simulink model "IEEE_religador"  (R2021b)
settings: Solver=ode23t  StartTime=0.0  StopTime=4  MaxStep=1e-4  RelTol=1e-3
undefined symbols (not defined in the file or in its folder): D1, Delta
libraries: spsThreePhasePISectionLineLib x36, spsThreePhaseVIMeasurementLib x34, spsSeriesRLCLoadLib x30, dsparch4 x24, spsSampleandHoldLib x24, spsNeutralLib x21, dspstat3 x20, spsPiSectionLineLib x15, spsLoadFlowBusLib x9, spsThreePhaseSeriesRLCLoadLib x8, spsThreePhaseFaultLib x7, spsThreePhaseBreakerLib x5
(part 1 of 2)
settings Model: SimulationMode=accelerator  Creator=Jamile-LARCA  LastModifiedBy=Ramayana
settings SolverCC: AlgebraicLoopSolver=TrustRegion
settings DataIOCC: ReturnWorkspaceOutputs=off
settings DebuggingCC: SFMachineParentedDataDiag=warning  ArithmeticOperatorsInVariantConditions=warning
settings SFSimCC: SimUseLocalCustomCode=off  CustomCodeUndefinedFunction=UseInterfaceOnly
settings RTWCC: RTWUseLocalCustomCode=off
settings CodeAppCC: StateflowObjectComments=on
settings SimscapeCC: SimscapeNormalizeSystem=off

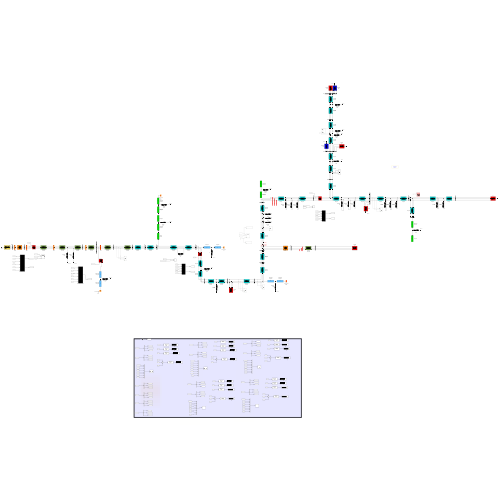
[thumbnail: Simulink's stored preview of the top-level diagram]
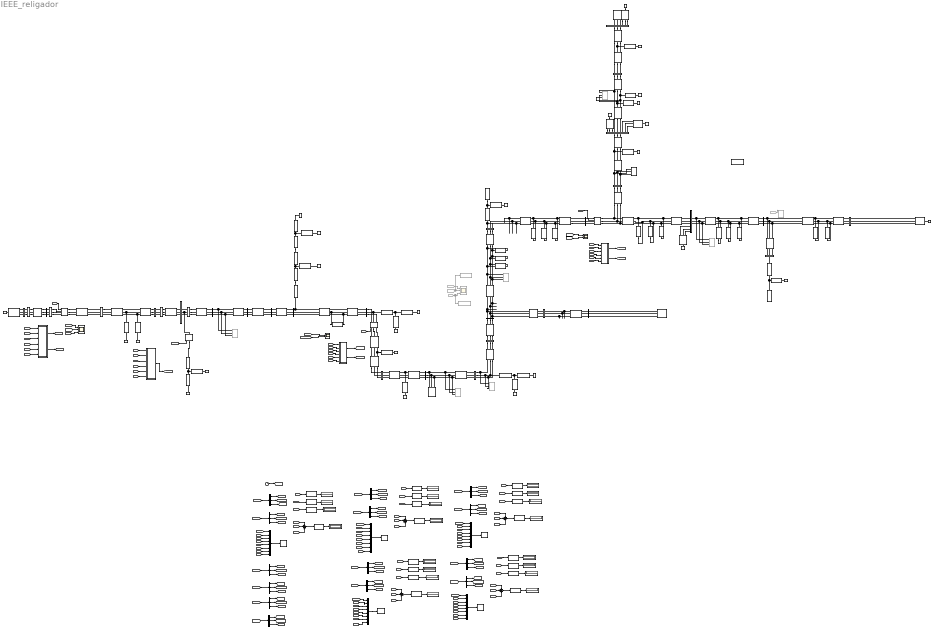
== system IEEE_religador ==
  note: 808
  note: Measurements
  " 816-824 D-I" : spsSeriesRLCLoadLib/Series RLC Load  LConnTagsString=a  RConnTagsString=__new0  NominalVoltage=24.9e3  NominalFrequency=60  ActivePower=5e3  InductivePower=2e3  CapacitivePower=0  Setx0=off  InitialVoltage=0  SetiL0=off  InitialCurrent=0  Measurements=None  LoadType=constant I
  " 824-826 Y-I" : spsSeriesRLCLoadLib/Series RLC Load  LConnTagsString=a  RConnTagsString=__new0  NominalVoltage=1.0156*14.376e3  NominalFrequency=60  ActivePower=40e3  InductivePower=20e3  CapacitivePower=0  Setx0=off  InitialVoltage=0  SetiL0=off  InitialCurrent=0  Measurements=None  LoadType=constant I
  " 828-830 Y-PQ" : spsSeriesRLCLoadLib/Series RLC Load  LConnTagsString=a  RConnTagsString=__new0  NominalVoltage=14.376e3  NominalFrequency=60  ActivePower=7e3  InductivePower=3e3  CapacitivePower=0  Setx0=off  InitialVoltage=0  SetiL0=off  InitialCurrent=0  Measurements=None  LoadType=constant PQ
  " 854-856 Y-PQ" : spsSeriesRLCLoadLib/Series RLC Load  LConnTagsString=a  RConnTagsString=__new0  NominalVoltage=0.9977*14.376e3  NominalFrequency=60  ActivePower=4e3  InductivePower=2e3  CapacitivePower=0  Setx0=off  InitialVoltage=0  SetiL0=off  InitialCurrent=0  Measurements=None  LoadType=constant PQ
  " L808-810a config 303 " : spsPiSectionLineLib/Pi Section Line  LConnTagsString=__new0  RConnTagsString=__new0  Phases=1  PiSections=1  Length=0.8845  Frequency=60  Resistance=1.7395  Inductance=2.4483e-3  Capacitance=6.9641e-9  Measurements=None  Measurements2=None
      settings: SourceProductBaseCode=PS
  " L808-810b config 303 " : spsPiSectionLineLib/Pi Section Line  LConnTagsString=__new0  RConnTagsString=__new0  Phases=1  PiSections=1  Length=0.8845  Frequency=60  Resistance=1.7395  Inductance=2.4483e-3  Capacitance=6.9641e-9  Measurements=None  Measurements2=None
      settings: SourceProductBaseCode=PS
  " L816-818 config 302" : spsPiSectionLineLib/Pi Section Line  LConnTagsString=__new0  RConnTagsString=__new0  Phases=1  PiSections=1  Length=0.521208  Frequency=60  Resistance=1.7395  Inductance=2.4483e-3  Capacitance=6.9641e-9  Measurements=None  Measurements2=None
      settings: SourceProductBaseCode=PS
  " L818-820a config 302" : spsPiSectionLineLib/Pi Section Line  LConnTagsString=__new0  RConnTagsString=__new0  Phases=1  PiSections=1  Length=7.3381  Frequency=60  Resistance=1.7395  Inductance=2.4483e-3  Capacitance=6.9641e-9  Measurements=None  Measurements2=None
      settings: SourceProductBaseCode=PS
  " L818-820b config 302" : spsPiSectionLineLib/Pi Section Line  LConnTagsString=__new0  RConnTagsString=__new0  Phases=1  PiSections=1  Length=7.3381  Frequency=60  Resistance=1.7395  Inductance=2.4483e-3  Capacitance=6.9641e-9  Measurements=None  Measurements2=None
      settings: SourceProductBaseCode=PS
  " L820-822a config 302" : spsPiSectionLineLib/Pi Section Line  LConnTagsString=__new0  RConnTagsString=__new0  Phases=1  PiSections=1  Length=2.0940  Frequency=60  Resistance=1.7395  Inductance=2.4483e-3  Capacitance=6.9641e-9  Measurements=None  Measurements2=None
      settings: SourceProductBaseCode=PS
  " L820-822b config 302" : spsPiSectionLineLib/Pi Section Line  LConnTagsString=__new0  RConnTagsString=__new0  Phases=1  PiSections=1  Length=2.0940  Frequency=60  Resistance=1.7395  Inductance=2.4483e-3  Capacitance=6.9641e-9  Measurements=None  Measurements2=None
      settings: SourceProductBaseCode=PS
  " L824-826a config 303 " : spsPiSectionLineLib/Pi Section Line  LConnTagsString=__new0  RConnTagsString=__new0  Phases=1  PiSections=1  Length=0.4618  Frequency=60  Resistance=1.7395  Inductance=2.4483e-3  Capacitance=6.9641e-9  Measurements=None  Measurements2=None
      settings: SourceProductBaseCode=PS
  " L824-826b config 303 " : spsPiSectionLineLib/Pi Section Line  LConnTagsString=__new0  RConnTagsString=__new0  Phases=1  PiSections=1  Length=0.4618  Frequency=60  Resistance=1.7395  Inductance=2.4483e-3  Capacitance=6.9641e-9  Measurements=None  Measurements2=None
      settings: SourceProductBaseCode=PS
  " L854-856a config 303 " : spsPiSectionLineLib/Pi Section Line  LConnTagsString=__new0  RConnTagsString=__new0  Phases=1  PiSections=1  Length=3.5555  Frequency=60  Resistance=1.7395  Inductance=2.4483e-3  Capacitance=6.9641e-9  Measurements=None  Measurements2=None
      settings: SourceProductBaseCode=PS
  " L854-856b config 303 " : spsPiSectionLineLib/Pi Section Line  LConnTagsString=__new0  RConnTagsString=__new0  Phases=1  PiSections=1  Length=3.5555  Frequency=60  Resistance=1.7395  Inductance=2.4483e-3  Capacitance=6.9641e-9  Measurements=None  Measurements2=None
      settings: SourceProductBaseCode=PS
  " L858-864a config 302" : spsPiSectionLineLib/Pi Section Line  LConnTagsString=__new0  RConnTagsString=__new0  Phases=1  PiSections=1  Length=0.2469  Frequency=60  Resistance=1.7395  Inductance=2.4483e-3  Capacitance=6.9641e-9  Measurements=None  Measurements2=None
      settings: SourceProductBaseCode=PS
  " L858-864b config 302" : spsPiSectionLineLib/Pi Section Line  LConnTagsString=__new0  RConnTagsString=__new0  Phases=1  PiSections=1  Length=0.2469  Frequency=60  Resistance=1.7395  Inductance=2.4483e-3  Capacitance=6.9641e-9  Measurements=None  Measurements2=None
      settings: SourceProductBaseCode=PS
  " L862-838a config 304" : spsPiSectionLineLib/Pi Section Line  LConnTagsString=__new0  RConnTagsString=__new0  Phases=1  PiSections=1  Length=0.7407  Frequency=60  Resistance=1.1941  Inductance=2.3425e-3  Capacitance=7.1925e-9  Measurements=None  Measurements2=None
      settings: SourceProductBaseCode=PS
  " L862-838b config 304" : spsPiSectionLineLib/Pi Section Line  LConnTagsString=__new0  RConnTagsString=__new0  Phases=1  PiSections=1  Length=0.7407  Frequency=60  Resistance=1.1941  Inductance=2.3425e-3  Capacitance=7.1925e-9  Measurements=None  Measurements2=None
      settings: SourceProductBaseCode=PS
  " Load 830 D-Z" : spsThreePhaseSeriesRLCLoadLib/Three-Phase Series RLC Load  LConnTagsString=A|B|C  Configuration=Delta  NominalVoltage=24.e3  Vabc=[1e3 1e3 1e3]  Vabcp=[24.9e3 24.9e3 24.9e3]  NominalFrequency=60  UnbalancedPower=on  ActivePower=450e3  InductivePower=225e3  CapacitivePower=0  Pabc=[10e3 9e3 11e3]  QLabc=[100 90 110]  QCabc=[100 90 110]  Pabcp=[10e3 10e3 25e3]  QLabcp=[5e3 5e3 10e3]  QCabcp=[0 0 0]  Measurements=None  LoadType=constant Z
  " Load 840 Y-I" : spsThreePhaseSeriesRLCLoadLib/Three-Phase Series RLC Load  LConnTagsString=A|B|C  RConnTagsString=N  Configuration=Y (neutral)  NominalVoltage=24.9e3  Vabc=[1e3 1e3 1e3]  Vabcp=[1e3 1e3 1e3]  NominalFrequency=60  UnbalancedPower=off  ActivePower=27e3  InductivePower=21e3  CapacitivePower=0  Pabc=[10e3 9e3 11e3]  QLabc=[100 90 110]  QCabc=[100 90 110]  Pabcp=[10e3 9e3 11e3]  QLabcp=[100 90 110]  QCabcp=[100 90 110]  Measurements=None  LoadType=constant I
  " Load 844 Y-Z" : spsThreePhaseSeriesRLCLoadLib/Three-Phase Series RLC Load  LConnTagsString=A|B|C  RConnTagsString=N  Configuration=Y (neutral)  NominalVoltage=24.9e3  Vabc=[1e3 1e3 1e3]  Vabcp=[1e3 1e3 1e3]  NominalFrequency=60  UnbalancedPower=off  ActivePower=405e3  InductivePower=315e3  CapacitivePower=0  Pabc=[10e3 9e3 11e3]  QLabc=[100 90 110]  QCabc=[100 90 110]  Pabcp=[10e3 9e3 11e3]  QLabcp=[100 90 110]  QCabcp=[100 90 110]  Measurements=None  LoadType=constant Z
  " Load 848 D-PQ" : spsThreePhaseSeriesRLCLoadLib/Three-Phase Series RLC Load  LConnTagsString=A|B|C  Configuration=Delta  NominalVoltage=24.9e3  Vabc=[1e3 1e3 1e3]  Vabcp=[1e3 1e3 1e3]  NominalFrequency=60  UnbalancedPower=off  ActivePower=60e3  InductivePower=48e3  CapacitivePower=0  Pabc=[10e3 9e3 11e3]  QLabc=[100 90 110]  QCabc=[100 90 110]  Pabcp=[10e3 9e3 11e3]  QLabcp=[100 90 110]  QCabcp=[100 90 110]  Measurements=None  LoadType=constant PQ
  " Load 860 Y-PQ" : spsThreePhaseSeriesRLCLoadLib/Three-Phase Series RLC Load  LConnTagsString=A|B|C  RConnTagsString=N  Configuration=Y (neutral)  NominalVoltage=24.9e3  Vabc=[1e3 1e3 1e3]  Vabcp=[1e3 1e3 1e3]  NominalFrequency=60  UnbalancedPower=off  ActivePower=60e3  InductivePower=48e3  CapacitivePower=0  Pabc=[10e3 9e3 11e3]  QLabc=[100 90 110]  QCabc=[100 90 110]  Pabcp=[10e3 9e3 11e3]  QLabcp=[100 90 110]  QCabcp=[100 90 110]  Measurements=None  LoadType=constant PQ
  " Load 890 D-I" : spsThreePhaseSeriesRLCLoadLib/Three-Phase Series RLC Load  LConnTagsString=A|B|C  Configuration=Delta  NominalVoltage=4.16e3  Vabc=[1e3 1e3 1e3]  Vabcp=[1e3 1e3 1e3]  NominalFrequency=60  UnbalancedPower=off  ActivePower=450e3  InductivePower=225e3  CapacitivePower=0  Pabc=[10e3 9e3 11e3]  QLabc=[100 90 110]  QCabc=[100 90 110]  Pabcp=[10e3 9e3 11e3]  QLabcp=[100 90 110]  QCabcp=[100 90 110]  Measurements=None  LoadType=constant I
  800 : spsThreePhaseVIMeasurementLib/Three-Phase V-I Measurement  VoltageMeasurement=phase-to-ground  SetLabelV=on  LabelV=Vabc_800  Vpu=off  VpuLL=off  CurrentMeasurement=yes  SetLabelI=on  LabelI=Iabc_800  Ipu=off  Pbase=100e6  Vbase=24.9e3  OutputType=Magnitude  PhasorSimulation=off  PSBequivalent=0
  802-806 b Y-PQ : spsSeriesRLCLoadLib/Series RLC Load  LConnTagsString=a  RConnTagsString=__new0  NominalVoltage=14.376e3  NominalFrequency=60  ActivePower=30e3  InductivePower=15e3  CapacitivePower=0  Setx0=off  InitialVoltage=0  SetiL0=off  InitialCurrent=0  Measurements=None  LoadType=constant PQ
  802-806 c Y-PQ : spsSeriesRLCLoadLib/Series RLC Load  LConnTagsString=a  RConnTagsString=__new0  NominalVoltage=14.376e3  NominalFrequency=60  ActivePower=25e3  InductivePower=14e3  CapacitivePower=0  Setx0=off  InitialVoltage=0  SetiL0=off  InitialCurrent=0  Measurements=None  LoadType=constant PQ
  806 : spsThreePhaseVIMeasurementLib/Three-Phase V-I Measurement  VoltageMeasurement=no  SetLabelV=on  LabelV=Vabc_806  Vpu=off  VpuLL=off  CurrentMeasurement=no  SetLabelI=on  LabelI=Iabc_806  Ipu=off  Pbase=100e6  Vbase=500e3  OutputType=Magnitude  PhasorSimulation=off  PSBequivalent=0
  808 : Subsystem
  812 : spsThreePhaseVIMeasurementLib/Three-Phase V-I Measurement  VoltageMeasurement=no  SetLabelV=on  LabelV=Vabc_812  Vpu=off  VpuLL=off  CurrentMeasurement=no  SetLabelI=on  LabelI=Iabc_812  Ipu=off  Pbase=100e6  Vbase=500e3  OutputType=Magnitude  PhasorSimulation=off  PSBequivalent=0
  814 : spsThreePhaseVIMeasurementLib/Three-Phase V-I Measurement  VoltageMeasurement=no  SetLabelV=on  LabelV=Vabc_814  Vpu=off  VpuLL=off  CurrentMeasurement=no  SetLabelI=on  LabelI=Iabc_814  Ipu=off  Pbase=100e6  Vbase=500e3  OutputType=Magnitude  PhasorSimulation=off  PSBequivalent=0
  816 : spsThreePhaseVIMeasurementLib/Three-Phase V-I Measurement  VoltageMeasurement=no  SetLabelV=on  LabelV=Vabc_816  Vpu=off  VpuLL=off  CurrentMeasurement=no  SetLabelI=on  LabelI=Iabc_816  Ipu=off  Pbase=100e6  Vbase=500e3  OutputType=Magnitude  PhasorSimulation=off  PSBequivalent=0
  818-820 Y-Z : spsSeriesRLCLoadLib/Series RLC Load  LConnTagsString=a  RConnTagsString=__new0  NominalVoltage=0.9926*14.376e3  NominalFrequency=60  ActivePower=34e3  InductivePower=17e3  CapacitivePower=0  Setx0=off  InitialVoltage=0  SetiL0=off  InitialCurrent=0  Measurements=None  LoadType=constant Z
  820-822 Y-PQ : spsSeriesRLCLoadLib/Series RLC Load  LConnTagsString=a  RConnTagsString=__new0  NominalVoltage=0.9895*14.376e3  NominalFrequency=60  ActivePower=135e3  InductivePower=70e3  CapacitivePower=0  Setx0=off  InitialVoltage=0  SetiL0=off  InitialCurrent=0  Measurements=None  LoadType=constant PQ
  824 : spsThreePhaseVIMeasurementLib/Three-Phase V-I Measurement  VoltageMeasurement=phase-to-ground  SetLabelV=on  LabelV=Vabc_824  Vpu=off  VpuLL=off  CurrentMeasurement=yes  SetLabelI=on  LabelI=Iabc_824  Ipu=off  Pbase=100e6  Vbase=500e3  OutputType=Magnitude  PhasorSimulation=off  PSBequivalent=0
  828 : spsThreePhaseVIMeasurementLib/Three-Phase V-I Measurement  VoltageMeasurement=no  SetLabelV=on  LabelV=Vabc_828  Vpu=off  VpuLL=off  CurrentMeasurement=no  SetLabelI=on  LabelI=Iabc_828  Ipu=off  Pbase=100e6  Vbase=500e3  OutputType=Magnitude  PhasorSimulation=off  PSBequivalent=0
  830 : spsThreePhaseVIMeasurementLib/Three-Phase V-I Measurement  VoltageMeasurement=no  SetLabelV=on  LabelV=Vabc_830  Vpu=off  VpuLL=off  CurrentMeasurement=no  SetLabelI=on  LabelI=Iabc_830  Ipu=off  Pbase=100e6  Vbase=500e3  OutputType=Magnitude  PhasorSimulation=off  PSBequivalent=0
  832 : spsThreePhaseVIMeasurementLib/Three-Phase V-I Measurement  VoltageMeasurement=phase-to-ground  SetLabelV=on  LabelV=Vabc_832  Vpu=off  VpuLL=off  CurrentMeasurement=yes  SetLabelI=on  LabelI=Iabc_832  Ipu=off  Pbase=100e6  Vbase=500e3  OutputType=Magnitude  PhasorSimulation=off  PSBequivalent=0
  832-858 D-Z : spsSeriesRLCLoadLib/Series RLC Load  LConnTagsString=a  RConnTagsString=__new0  NominalVoltage=24.9e3  NominalFrequency=60  ActivePower=6e3  InductivePower=3e3  CapacitivePower=0  Setx0=off  InitialVoltage=0  SetiL0=off  InitialCurrent=0  Measurements=None  LoadType=constant Z
  832-858a D-Z : spsSeriesRLCLoadLib/Series RLC Load  LConnTagsString=a  RConnTagsString=__new0  NominalVoltage=24.9e3  NominalFrequency=60  ActivePower=7e3  InductivePower=3e3  CapacitivePower=0  Setx0=off  InitialVoltage=0  SetiL0=off  InitialCurrent=0  Measurements=None  LoadType=constant Z
  832-858b D-Z : spsSeriesRLCLoadLib/Series RLC Load  LConnTagsString=a  RConnTagsString=__new0  NominalVoltage=24.9e3  NominalFrequency=60  ActivePower=2e3  InductivePower=1e3  CapacitivePower=0  Setx0=off  InitialVoltage=0  SetiL0=off  InitialCurrent=0  Measurements=None  LoadType=constant Z
  834 : spsThreePhaseVIMeasurementLib/Three-Phase V-I Measurement  VoltageMeasurement=phase-to-ground  SetLabelV=on  LabelV=Vabc_834  Vpu=off  VpuLL=off  CurrentMeasurement=yes  SetLabelI=on  LabelI=Iabc_834  Ipu=off  Pbase=100e6  Vbase=500e3  OutputType=Magnitude  PhasorSimulation=off  PSBequivalent=0
  834-860a D-Z : spsSeriesRLCLoadLib/Series RLC Load  LConnTagsString=a  RConnTagsString=__new0  NominalVoltage=24.9e3  NominalFrequency=60  ActivePower=16e3  InductivePower=8e3  CapacitivePower=0  Setx0=off  InitialVoltage=0  SetiL0=off  InitialCurrent=0  Measurements=None  LoadType=constant Z
  834-860b D-Z : spsSeriesRLCLoadLib/Series RLC Load  LConnTagsString=a  RConnTagsString=__new0  NominalVoltage=24.9e3  NominalFrequency=60  ActivePower=20e3  InductivePower=10e3  CapacitivePower=0  Setx0=off  InitialVoltage=0  SetiL0=off  InitialCurrent=0  Measurements=None  LoadType=constant Z
  834-860c D-Z : spsSeriesRLCLoadLib/Series RLC Load  LConnTagsString=a  RConnTagsString=__new0  NominalVoltage=24.9e3  NominalFrequency=60  ActivePower=110e3  InductivePower=55e3  CapacitivePower=0  Setx0=off  InitialVoltage=0  SetiL0=off  InitialCurrent=0  Measurements=None  LoadType=constant Z
  836 : spsThreePhaseVIMeasurementLib/Three-Phase V-I Measurement  VoltageMeasurement=phase-to-ground  SetLabelV=on  LabelV=Vabc_836  Vpu=off  VpuLL=off  CurrentMeasurement=yes  SetLabelI=on  LabelI=Iabc_836  Ipu=off  Pbase=100e6  Vbase=500e3  OutputType=Magnitude  PhasorSimulation=off  PSBequivalent=0
  836-840a D-I : spsSeriesRLCLoadLib/Series RLC Load  LConnTagsString=a  RConnTagsString=__new0  NominalVoltage=24.9e3  NominalFrequency=60  ActivePower=18e3  InductivePower=9e3  CapacitivePower=0  Setx0=off  InitialVoltage=0  SetiL0=off  InitialCurrent=0  Measurements=None  LoadType=constant I
  836-840b D-I : spsSeriesRLCLoadLib/Series RLC Load  LConnTagsString=a  RConnTagsString=__new0  NominalVoltage=24.9e3  NominalFrequency=60  ActivePower=22e3  InductivePower=11e3  CapacitivePower=0  Setx0=off  InitialVoltage=0  SetiL0=off  InitialCurrent=0  Measurements=None  LoadType=constant I
  840 : spsThreePhaseVIMeasurementLib/Three-Phase V-I Measurement  VoltageMeasurement=phase-to-ground  SetLabelV=on  LabelV=Vabc_840  Vpu=off  VpuLL=off  CurrentMeasurement=yes  SetLabelI=on  LabelI=Iabc_840  Ipu=off  Pbase=100e6  Vbase=500e3  OutputType=Magnitude  PhasorSimulation=off  PSBequivalent=0
  842 : spsThreePhaseVIMeasurementLib/Three-Phase V-I Measurement  VoltageMeasurement=phase-to-ground  SetLabelV=on  LabelV=Vabc_842  Vpu=off  VpuLL=off  CurrentMeasurement=yes  SetLabelI=on  LabelI=Iabc_842  Ipu=off  Pbase=100e6  Vbase=500e3  OutputType=Magnitude  PhasorSimulation=off  PSBequivalent=0
  842-844 Y-PQ : spsSeriesRLCLoadLib/Series RLC Load  LConnTagsString=a  RConnTagsString=__new0  NominalVoltage=14.376e3  NominalFrequency=60  ActivePower=9e3  InductivePower=5e3  CapacitivePower=0  Setx0=off  InitialVoltage=0  SetiL0=off  InitialCurrent=0  Measurements=None  LoadType=constant PQ
  844 : Subsystem
  844-846b Y-PQ : spsSeriesRLCLoadLib/Series RLC Load  LConnTagsString=a  RConnTagsString=__new0  NominalVoltage=14.376e3  NominalFrequency=60  ActivePower=25e3  InductivePower=12e3  CapacitivePower=0  Setx0=off  InitialVoltage=0  SetiL0=off  InitialCurrent=0  Measurements=None  LoadType=constant PQ
  844-846c Y-PQ2 : spsSeriesRLCLoadLib/Series RLC Load  LConnTagsString=a  RConnTagsString=__new0  NominalVoltage=14.376e3  NominalFrequency=60  ActivePower=20e3  InductivePower=11e3  CapacitivePower=0  Setx0=off  InitialVoltage=0  SetiL0=off  InitialCurrent=0  Measurements=None  LoadType=constant PQ
  846 : spsThreePhaseVIMeasurementLib/Three-Phase V-I Measurement  VoltageMeasurement=no  SetLabelV=on  LabelV=Vabc_846  Vpu=off  VpuLL=off  CurrentMeasurement=no  SetLabelI=on  LabelI=Iabc_846  Ipu=off  Pbase=100e6  Vbase=500e3  OutputType=Magnitude  PhasorSimulation=off  PSBequivalent=0
  846-848b Y-PQ : spsSeriesRLCLoadLib/Series RLC Load  LConnTagsString=a  RConnTagsString=__new0  NominalVoltage=14.376e3  NominalFrequency=60  ActivePower=23e3  InductivePower=11e3  CapacitivePower=0  Setx0=off  InitialVoltage=0  SetiL0=off  InitialCurrent=0  Measurements=None  LoadType=constant PQ
  848 : Subsystem
  850 : spsThreePhaseVIMeasurementLib/Three-Phase V-I Measurement  VoltageMeasurement=no  SetLabelV=on  LabelV=Vabc_850  Vpu=off  VpuLL=off  CurrentMeasurement=no  SetLabelI=on  LabelI=Iabc_850  Ipu=off  Pbase=100e6  Vbase=500e3  OutputType=Magnitude  PhasorSimulation=off  PSBequivalent=0
  852 : spsThreePhaseVIMeasurementLib/Three-Phase V-I Measurement  VoltageMeasurement=no  SetLabelV=on  LabelV=Vabc_852  Vpu=off  VpuLL=off  CurrentMeasurement=no  SetLabelI=on  LabelI=Iabc_852  Ipu=off  Pbase=100e6  Vbase=500e3  OutputType=Magnitude  PhasorSimulation=off  PSBequivalent=0
  854 : spsThreePhaseVIMeasurementLib/Three-Phase V-I Measurement  VoltageMeasurement=no  SetLabelV=on  LabelV=Vabc_854  Vpu=off  VpuLL=off  CurrentMeasurement=no  SetLabelI=on  LabelI=Iabc_854  Ipu=off  Pbase=100e6  Vbase=500e3  OutputType=Magnitude  PhasorSimulation=off  PSBequivalent=0
  858 : spsThreePhaseVIMeasurementLib/Three-Phase V-I Measurement  VoltageMeasurement=no  SetLabelV=on  LabelV=Vabc_858  Vpu=off  VpuLL=off  CurrentMeasurement=no  SetLabelI=on  LabelI=Iabc_858  Ipu=off  Pbase=100e6  Vbase=500e3  OutputType=Magnitude  PhasorSimulation=off  PSBequivalent=0
  858-834a D-PQ : spsSeriesRLCLoadLib/Series RLC Load  LConnTagsString=a  RConnTagsString=__new0  NominalVoltage=24.9e3  NominalFrequency=60  ActivePower=4e3  InductivePower=2e3  CapacitivePower=0  Setx0=off  InitialVoltage=0  SetiL0=off  InitialCurrent=0  Measurements=None  LoadType=constant PQ
  858-834b D-PQ : spsSeriesRLCLoadLib/Series RLC Load  LConnTagsString=a  RConnTagsString=__new0  NominalVoltage=24.9e3  NominalFrequency=60  ActivePower=15e3  InductivePower=8e3  CapacitivePower=0  Setx0=off  InitialVoltage=0  SetiL0=off  InitialCurrent=0  Measurements=None  LoadType=constant PQ
  858-834c D-PQ : spsSeriesRLCLoadLib/Series RLC Load  LConnTagsString=a  RConnTagsString=__new0  NominalVoltage=24.9e3  NominalFrequency=60  ActivePower=13e3  InductivePower=7e3  CapacitivePower=0  Setx0=off  InitialVoltage=0  SetiL0=off  InitialCurrent=0  Measurements=None  LoadType=constant PQ
  858-864 Y-PQ : spsSeriesRLCLoadLib/Series RLC Load  LConnTagsString=a  RConnTagsString=__new0  NominalVoltage=14.376e3  NominalFrequency=60  ActivePower=2e3  InductivePower=1e3  CapacitivePower=0  Setx0=off  InitialVoltage=0  SetiL0=off  InitialCurrent=0  Measurements=None  LoadType=constant PQ
  860 : Subsystem
  860-836a D-PQ : spsSeriesRLCLoadLib/Series RLC Load  LConnTagsString=a  RConnTagsString=__new0  NominalVoltage=24.9e3  NominalFrequency=60  ActivePower=30e3  InductivePower=15e3  CapacitivePower=0  Setx0=off  InitialVoltage=0  SetiL0=off  InitialCurrent=0  Measurements=None  LoadType=constant PQ
  860-836b D-PQ : spsSeriesRLCLoadLib/Series RLC Load  LConnTagsString=a  RConnTagsString=__new0  NominalVoltage=24.9e3  NominalFrequency=60  ActivePower=10e3  InductivePower=6e3  CapacitivePower=0  Setx0=off  InitialVoltage=0  SetiL0=off  InitialCurrent=0  Measurements=None  LoadType=constant PQ
  860-836c D-PQ : spsSeriesRLCLoadLib/Series RLC Load  LConnTagsString=a  RConnTagsString=__new0  NominalVoltage=24.9e3  NominalFrequency=60  ActivePower=42e3  InductivePower=22e3  CapacitivePower=0  Setx0=off  InitialVoltage=0  SetiL0=off  InitialCurrent=0  Measurements=None  LoadType=constant PQ
  862 : spsThreePhaseVIMeasurementLib/Three-Phase V-I Measurement  VoltageMeasurement=no  SetLabelV=on  LabelV=Vabc_862  Vpu=off  VpuLL=off  CurrentMeasurement=no  SetLabelI=on  LabelI=Iabc_862  Ipu=off  Pbase=100e6  Vbase=500e3  OutputType=Magnitude  PhasorSimulation=off  PSBequivalent=0
  862-838 Y-PQ : spsSeriesRLCLoadLib/Series RLC Load  LConnTagsString=a  RConnTagsString=__new0  NominalVoltage=14.376e3  NominalFrequency=60  ActivePower=28e3  InductivePower=14e3  CapacitivePower=0  Setx0=off  InitialVoltage=0  SetiL0=off  InitialCurrent=0  Measurements=None  LoadType=constant PQ
  888 : spsThreePhaseVIMeasurementLib/Three-Phase V-I Measurement  VoltageMeasurement=no  SetLabelV=on  LabelV=Vabc_888  Vpu=off  VpuLL=off  CurrentMeasurement=no  SetLabelI=on  LabelI=Iabc_888  Ipu=off  Pbase=100e6  Vbase=500e3  OutputType=Magnitude  PhasorSimulation=off  PSBequivalent=0
  890 : spsThreePhaseVIMeasurementLib/Three-Phase V-I Measurement  VoltageMeasurement=no  SetLabelV=on  LabelV=Vabc_890  Vpu=off  VpuLL=off  CurrentMeasurement=no  SetLabelI=on  LabelI=Iabc_890  Ipu=off  Pbase=100e6  Vbase=500e3  OutputType=Magnitude  PhasorSimulation=off  PSBequivalent=0
  BSUB : spsThreePhaseVIMeasurementLib/Three-Phase V-I Measurement  VoltageMeasurement=no  SetLabelV=on  LabelV=Vabc_SUB  Vpu=off  VpuLL=off  CurrentMeasurement=no  SetLabelI=on  LabelI=Iabc_SUB  Ipu=off  Pbase=100e6  Vbase=500e3  OutputType=Magnitude  PhasorSimulation=off  PSBequivalent=0
  Bus Creator{1,3..6} (5 alike) : BusCreator  Inputs=8
  Capacitor 848 : spsThreePhaseSeriesRLCLoadLib/Three-Phase Series RLC Load  LConnTagsString=A|B|C  RConnTagsString=N  Configuration=Y (neutral)  NominalVoltage=24.9e3  Vabc=[1e3 1e3 1e3]  Vabcp=[1e3 1e3 1e3]  NominalFrequency=60  UnbalancedPower=off  ActivePower=0  InductivePower=0  CapacitivePower=450e3  Pabc=[10e3 9e3 11e3]  QLabc=[100 90 110]  QCabc=[100 90 110]  Pabcp=[10e3 9e3 11e3]  QLabcp=[100 90 110]  QCabcp=[100 90 110]  Measurements=None  LoadType=constant Z
  Capacitor 844 : spsThreePhaseSeriesRLCLoadLib/Three-Phase Series RLC Load  LConnTagsString=A|B|C  RConnTagsString=N  Configuration=Y (neutral)  NominalVoltage=24.9e3  Vabc=[1e3 1e3 1e3]  Vabcp=[1e3 1e3 1e3]  NominalFrequency=60  UnbalancedPower=off  ActivePower=0  InductivePower=0  CapacitivePower=300e3  Pabc=[10e3 9e3 11e3]  QLabc=[100 90 110]  QCabc=[100 90 110]  Pabcp=[10e3 9e3 11e3]  QLabcp=[100 90 110]  QCabcp=[100 90 110]  Measurements=None  LoadType=constant Z
  Clock1 : Clock
  Demux{1..14} (14 alike) : Demux  Outputs=3
  From179 : From  Commented=on  GotoTag=Vabc_832  TagVisibility=global
  From180 : From  Commented=on  GotoTag=Iabc_832  TagVisibility=global
  From181 : From  Commented=on  GotoTag=Trp832
  From45 : From  Commented=on  GotoTag=Trip836
  Ia{1,3..5} (4 alike) : Display
  Ia_1 : Display
  Ib{1,3..5} (4 alike) : Display
  Ib_1 : Display
  Ic{1,3..5} (4 alike) : Display
  Ic_1 : Display
  "In3 " : Display
  "In4 " : Display
  In4 1 : Display
  In4 2 : Display
  "In_1 " : Display
  L800-802 config 300 : spsThreePhasePISectionLineLib/Three-Phase PI Section Line  LConnTagsString=a|b|c  RConnTagsString=A|B|C  Length=0.786384  Frequency=60  Resistances=[ 0.6960 1.0873]  Inductances="[ 1.3735e-3  3.9091e-3]"  Capacitances=[10.1464e-9 4.9598e-9]
  L802-806a config 300 : spsThreePhasePISectionLineLib/Three-Phase PI Section Line  LConnTagsString=a|b|c  RConnTagsString=A|B|C  Length=0.2637  Frequency=60  Resistances=[ 0.6960 1.0873]  Inductances="[ 1.3735e-3  3.9091e-3]"  Capacitances=[10.1464e-9 4.9598e-9]
  L802-806b config 300 : spsThreePhasePISectionLineLib/Three-Phase PI Section Line  LConnTagsString=a|b|c  RConnTagsString=A|B|C  Length=0.2637  Frequency=60  Resistances=[ 0.6960 1.0873]  Inductances="[ 1.3735e-3  3.9091e-3]"  Capacitances=[10.1464e-9 4.9598e-9]
  L806-808 config 300 : spsThreePhasePISectionLineLib/Three-Phase PI Section Line  LConnTagsString=a|b|c  RConnTagsString=A|B|C  Length=9.823704  Frequency=60  Resistances=[ 0.6960 1.0873]  Inductances="[ 1.3735e-3  3.9091e-3]"  Capacitances=[10.1464e-9 4.9598e-9]
  L808-812 config 300 : spsThreePhasePISectionLineLib/Three-Phase PI Section Line  LConnTagsString=a|b|c  RConnTagsString=A|B|C  Length=11.43  Frequency=60  Resistances=[ 0.6960 1.0873]  Inductances="[ 1.3735e-3  3.9091e-3]"  Capacitances=[10.1464e-9 4.9598e-9]
  L812-814 config 300 : spsThreePhasePISectionLineLib/Three-Phase PI Section Line  LConnTagsString=a|b|c  RConnTagsString=A|B|C  Length=9.061704  Frequency=60  Resistances=[ 0.6960 1.0873]  Inductances="[ 1.3735e-3  3.9091e-3]"  Capacitances=[10.1464e-9 4.9598e-9]
  L814-850 config 301 : spsThreePhasePISectionLineLib/Three-Phase PI Section Line  LConnTagsString=a|b|c  RConnTagsString=A|B|C  Length=0.003048  Frequency=60  Resistances=[ 1.0502 1.4835]  Inductances="[ 1.3865e-3  4.2494e-3]"  Capacitances=[9.7318e-9 4.8338e-9]
  L816-824a config 301 : spsThreePhasePISectionLineLib/Three-Phase PI Section Line  LConnTagsString=a|b|c  RConnTagsString=A|B|C  Length=1.5560  Frequency=60  Resistances=[ 1.0502 1.4835]  Inductances="[ 1.3865e-3  4.2494e-3]"  Capacitances=[9.7318e-9 4.8338e-9]
  L816-824b config 301 : spsThreePhasePISectionLineLib/Three-Phase PI Section Line  LConnTagsString=a|b|c  RConnTagsString=A|B|C  Length=1.5560  Frequency=60  Resistances=[ 1.0502 1.4835]  Inductances="[ 1.3865e-3  4.2494e-3]"  Capacitances=[9.7318e-9 4.8338e-9]
  L824-828a config 301 : spsThreePhasePISectionLineLib/Three-Phase PI Section Line  LConnTagsString=a|b|c  RConnTagsString=A|B|C  Length=0.1280  Frequency=60  Resistances=[ 1.0502 1.4835]  Inductances="[ 1.3865e-3  4.2494e-3]"  Capacitances=[9.7318e-9 4.8338e-9]
  L824-828b config 301 : spsThreePhasePISectionLineLib/Three-Phase PI Section Line  LConnTagsString=a|b|c  RConnTagsString=A|B|C  Length=0.1280  Frequency=60  Resistances=[ 1.0502 1.4835]  Inductances="[ 1.3865e-3  4.2494e-3]"  Capacitances=[9.7318e-9 4.8338e-9]
  L828-830a config 301 : spsThreePhasePISectionLineLib/Three-Phase PI Section Line  LConnTagsString=a|b|c  RConnTagsString=A|B|C  Length=3.1151  Frequency=60  Resistances=[ 1.0502 1.4835]  Inductances="[ 1.3865e-3  4.2494e-3]"  Capacitances=[9.7318e-9 4.8338e-9]
  L828-830b config 301 : spsThreePhasePISectionLineLib/Three-Phase PI Section Line  LConnTagsString=a|b|c  RConnTagsString=A|B|C  Length=3.1151  Frequency=60  Resistances=[ 1.0502 1.4835]  Inductances="[ 1.3865e-3  4.2494e-3]"  Capacitances=[9.7318e-9 4.8338e-9]
  L830-854 config 301 : spsThreePhasePISectionLineLib/Three-Phase PI Section Line  LConnTagsString=a|b|c  RConnTagsString=A|B|C  Length=0.158496  Frequency=60  Resistances=[ 1.0502 1.4835]  Inductances="[ 1.3865e-3  4.2494e-3]"  Capacitances=[9.7318e-9 4.8338e-9]
  L832-858a config 301 : spsThreePhasePISectionLineLib/Three-Phase PI Section Line  LConnTagsString=a|b|c  RConnTagsString=A|B|C  Length=0.74676  Frequency=60  Resistances=[ 1.0502 1.4835]  Inductances="[ 1.3865e-3  4.2494e-3]"  Capacitances=[9.7318e-9 4.8338e-9]
  L832-858b config 301 : spsThreePhasePISectionLineLib/Three-Phase PI Section Line  LConnTagsString=a|b|c  RConnTagsString=A|B|C  Length=0.74676  Frequency=60  Resistances=[ 1.0502 1.4835]  Inductances="[ 1.3865e-3  4.2494e-3]"  Capacitances=[9.7318e-9 4.8338e-9]
  L834-842 config 301 : spsThreePhasePISectionLineLib/Three-Phase PI Section Line  LConnTagsString=a|b|c  RConnTagsString=A|B|C  Length=0.085344  Frequency=60  Resistances=[ 1.0502 1.4835]  Inductances="[ 1.3865e-3  4.2494e-3]"  Capacitances=[9.7318e-9 4.8338e-9]
  L834-860a config 301 : spsThreePhasePISectionLineLib/Three-Phase PI Section Line  LConnTagsString=a|b|c  RConnTagsString=A|B|C  Length=0.3078  Frequency=60  Resistances=[ 1.0502 1.4835]  Inductances="[ 1.3865e-3  4.2494e-3]"  Capacitances=[9.7318e-9 4.8338e-9]
  L834-860b config 301 : spsThreePhasePISectionLineLib/Three-Phase PI Section Line  LConnTagsString=a|b|c  RConnTagsString=A|B|C  Length=0.3078  Frequency=60  Resistances=[ 1.0502 1.4835]  Inductances="[ 1.3865e-3  4.2494e-3]"  Capacitances=[9.7318e-9 4.8338e-9]
  L836-840a config 301 : spsThreePhasePISectionLineLib/Three-Phase PI Section Line  LConnTagsString=a|b|c  RConnTagsString=A|B|C  Length=0.1311  Frequency=60  Resistances=[ 1.0502 1.4835]  Inductances="[ 1.3865e-3  4.2494e-3]"  Capacitances=[9.7318e-9 4.8338e-9]
  L836-840b config 301 : spsThreePhasePISectionLineLib/Three-Phase PI Section Line  LConnTagsString=a|b|c  RConnTagsString=A|B|C  Length=0.1311  Frequency=60  Resistances=[ 1.0502 1.4835]  Inductances="[ 1.3865e-3  4.2494e-3]"  Capacitances=[9.7318e-9 4.8338e-9]
  L836-862 config 301 : spsThreePhasePISectionLineLib/Three-Phase PI Section Line  LConnTagsString=a|b|c  RConnTagsString=A|B|C  Length=0.085344  Frequency=60  Resistances=[ 1.0502 1.4835]  Inductances="[ 1.3865e-3  4.2494e-3]"  Capacitances=[9.7318e-9 4.8338e-9]
  L842-844a config 301 : spsThreePhasePISectionLineLib/Three-Phase PI Section Line  LConnTagsString=a|b|c  RConnTagsString=A|B|C  Length=0.2057  Frequency=60  Resistances=[ 1.0502 1.4835]  Inductances="[ 1.3865e-3  4.2494e-3]"  Capacitances=[9.7318e-9 4.8338e-9]
  L842-844b config 301 : spsThreePhasePISectionLineLib/Three-Phase PI Section Line  LConnTagsString=a|b|c  RConnTagsString=A|B|C  Length=0.2057  Frequency=60  Resistances=[ 1.0502 1.4835]  Inductances="[ 1.3865e-3  4.2494e-3]"  Capacitances=[9.7318e-9 4.8338e-9]
  L844-846a config 301 : spsThreePhasePISectionLineLib/Three-Phase PI Section Line  LConnTagsString=a|b|c  RConnTagsString=A|B|C  Length=0.5547  Frequency=60  Resistances=[ 1.0502 1.4835]  Inductances="[ 1.3865e-3  4.2494e-3]"  Capacitances=[9.7318e-9 4.8338e-9]
  L844-846b config 301 : spsThreePhasePISectionLineLib/Three-Phase PI Section Line  LConnTagsString=a|b|c  RConnTagsString=A|B|C  Length=0.5547  Frequency=60  Resistances=[ 1.0502 1.4835]  Inductances="[ 1.3865e-3  4.2494e-3]"  Capacitances=[9.7318e-9 4.8338e-9]
  L846-848a config 301 : spsThreePhasePISectionLineLib/Three-Phase PI Section Line  LConnTagsString=a|b|c  RConnTagsString=A|B|C  Length=0.0808  Frequency=60  Resistances=[ 1.0502 1.4835]  Inductances="[ 1.3865e-3  4.2494e-3]"  Capacitances=[9.7318e-9 4.8338e-9]
  L846-848b config 301 : spsThreePhasePISectionLineLib/Three-Phase PI Section Line  LConnTagsString=a|b|c  RConnTagsString=A|B|C  Length=0.0808  Frequency=60  Resistances=[ 1.0502 1.4835]  Inductances="[ 1.3865e-3  4.2494e-3]"  Capacitances=[9.7318e-9 4.8338e-9]
  L850-816 config 301 : spsThreePhasePISectionLineLib/Three-Phase PI Section Line  LConnTagsString=a|b|c  RConnTagsString=A|B|C  Length=0.094488  Frequency=60  Resistances=[ 1.0502 1.4835]  Inductances="[ 1.3865e-3  4.2494e-3]"  Capacitances=[9.7318e-9 4.8338e-9]
  L852-832 config 301 : spsThreePhasePISectionLineLib/Three-Phase PI Section Line  LConnTagsString=a|b|c  RConnTagsString=A|B|C  Length=0.003048  Frequency=60  Resistances=[ 1.0502 1.4835]  Inductances="[ 1.3865e-3  4.2494e-3]"  Capacitances=[9.7318e-9 4.8338e-9]
  L854-852 config 301 : spsThreePhasePISectionLineLib/Three-Phase PI Section Line  LConnTagsString=a|b|c  RConnTagsString=A|B|C  Length=11.225784  Frequency=60  Resistances=[ 1.0502 1.4835]  Inductances="[ 1.3865e-3  4.2494e-3]"  Capacitances=[9.7318e-9 4.8338e-9]
  L858-834a config 301 : spsThreePhasePISectionLineLib/Three-Phase PI Section Line  LConnTagsString=a|b|c  RConnTagsString=A|B|C  Length=0.8885  Frequency=60  Resistances=[ 1.0502 1.4835]  Inductances="[ 1.3865e-3  4.2494e-3]"  Capacitances=[9.7318e-9 4.8338e-9]
  L858-834b config 301 : spsThreePhasePISectionLineLib/Three-Phase PI Section Line  LConnTagsString=a|b|c  RConnTagsString=A|B|C  Length=0.8885  Frequency=60  Resistances=[ 1.0502 1.4835]  Inductances="[ 1.3865e-3  4.2494e-3]"  Capacitances=[9.7318e-9 4.8338e-9]
  L860-836a config 301 : spsThreePhasePISectionLineLib/Three-Phase PI Section Line  LConnTagsString=a|b|c  RConnTagsString=A|B|C  Length=0.4084  Frequency=60  Resistances=[ 1.0502 1.4835]  Inductances="[ 1.3865e-3  4.2494e-3]"  Capacitances=[9.7318e-9 4.8338e-9]
  L860-836b config 301 : spsThreePhasePISectionLineLib/Three-Phase PI Section Line  LConnTagsString=a|b|c  RConnTagsString=A|B|C  Length=0.4084  Frequency=60  Resistances=[ 1.0502 1.4835]  Inductances="[ 1.3865e-3  4.2494e-3]"  Capacitances=[9.7318e-9 4.8338e-9]
  L888-890 config 300 : spsThreePhasePISectionLineLib/Three-Phase PI Section Line  LConnTagsString=a|b|c  RConnTagsString=A|B|C  Length=3.218688  Frequency=60  Resistances=[ 0.6960 1.0873]  Inductances="[ 1.3735e-3  3.9091e-3]"  Capacitances=[10.1464e-9 4.9598e-9]
  Load 808-810 Y-I : spsSeriesRLCLoadLib/Series RLC Load  LConnTagsString=a  RConnTagsString=__new0  NominalVoltage=14.376e3  NominalFrequency=60  ActivePower=16e3  InductivePower=8e3  CapacitivePower=0  Setx0=off  InitialVoltage=0  SetiL0=off  InitialCurrent=0  Measurements=None  LoadType=constant I
  Load 824-828 Y-PQ : spsSeriesRLCLoadLib/Series RLC Load  LConnTagsString=a  RConnTagsString=__new0  NominalVoltage=1.0109*14.376e3  NominalFrequency=60  ActivePower=4e3  InductivePower=2e3  CapacitivePower=0  Setx0=off  InitialVoltage=0  SetiL0=off  InitialCurrent=0  Measurements=None  LoadType=constant PQ
  Load Flow Bar : spsLoadFlowBusLib/Load Flow Bus  LConnTagsString=a|b|c  RConnTagsString=a|b|c  Phases=ABC  Connectors=on both sides  ID=SUB  Vbase=69e3/sqrt(3)  Vref="[ 1.05  1.05  1.05]"  Vangle="[ 0.00  -120.00  120.00]"  VLF=1.021  VLFb=1.042  VLFc=1.017  angleLF=-2.49  angleLFb=-121.7  angleLFc=117.8
      settings: AttributesFormatString=%<ID>  SourceProductBaseCode=PS
  Load Flow Bar1 : spsLoadFlowBusLib/Load Flow Bus  LConnTagsString=a|b|c  RConnTagsString=a|b|c  Phases=ABC  Connectors=on both sides  ID=800  Vbase=24.9e3/sqrt(3)  Vref="[ 1.05  1.05  1.05]"  Vangle="[ 0.00  -120.00  120.00]"  VLF=1.021  VLFb=1.042  VLFc=1.017  angleLF=-2.49  angleLFb=-121.7  angleLFc=117.8
      settings: AttributesFormatString=%<ID>  SourceProductBaseCode=PS
  Load Flow Bar2 : spsLoadFlowBusLib/Load Flow Bus  LConnTagsString=a|b|c  RConnTagsString=a|b|c  Phases=ABC  Connectors=on both sides  ID=802  Vbase=24.9e3/sqrt(3)  Vref="[ 1.0475  1.0484  1.0484]"  Vangle="[ -0.05  -120.07  119.95]"  VLF=1.021  VLFb=1.042  VLFc=1.017  angleLF=-2.49  angleLFb=-121.7  angleLFc=117.8
      settings: AttributesFormatString=%<ID>  SourceProductBaseCode=PS
  Load Flow Bar3 : spsLoadFlowBusLib/Load Flow Bus  LConnTagsString=a|b|c  RConnTagsString=a|b|c  Phases=ABC  Connectors=on both sides  ID=806  Vbase=24.9e3/sqrt(3)  Vref="[ 1.0457  1.0474  1.0474]"  Vangle="[ -0.08  -120.11  119.92]"  VLF=1.021  VLFb=1.042  VLFc=1.017  angleLF=-2.49  angleLFb=-121.7  angleLFc=117.8
      settings: AttributesFormatString=%<ID>  SourceProductBaseCode=PS
  Load Flow Bar4 : spsLoadFlowBusLib/Load Flow Bus  LConnTagsString=a|b|c  RConnTagsString=a|b|c  Phases=ABC  Connectors=on both sides  ID=808  Vbase=24.9e3/sqrt(3)  Vref="[ 1.0136  1.0296  1.0289]"  Vangle="[ -0.75  -120.95  119.30]"  VLF=1.021  VLFb=1.042  VLFc=1.017  angleLF=-2.49  angleLFb=-121.7  angleLFc=117.8
      settings: AttributesFormatString=%<ID>  SourceProductBaseCode=PS
  Load Flow Bus : spsLoadFlowBusLib/Load Flow Bus  LConnTagsString=a  Phases=B  Connectors=on one side  ID=810  Vbase=24.9e3/sqrt(3)  Vref=1.00  Vangle=0  VLF=1  VLFb=1  VLFc=1  angleLF=0  angleLFb=0  angleLFc=0
      settings: SourceProductBaseCode=PS
  Load Flow Bus1 : spsLoadFlowBusLib/Load Flow Bus  LConnTagsString=a  Phases=A  Connectors=on one side  ID=822  Vbase=24.9e3/sqrt(3)  Vref=1  Vangle=0.0  VLF=1  VLFb=1  VLFc=1  angleLF=0  angleLFb=0  angleLFc=0
      settings: SourceProductBaseCode=PS
  Load Flow Bus2 : spsLoadFlowBusLib/Load Flow Bus  LConnTagsString=a  Phases=B  Connectors=on one side  ID=826  Vbase=24.9e3/sqrt(3)  Vref=1  Vangle=0  VLF=1  VLFb=1  VLFc=1  angleLF=0  angleLFb=0  angleLFc=0
      settings: SourceProductBaseCode=PS
  Load Flow Bus3 : spsLoadFlowBusLib/Load Flow Bus  LConnTagsString=a  Phases=B  Connectors=on one side  ID=856  Vbase=24.9e3/sqrt(3)  Vref=1  Vangle=0  VLF=1  VLFb=1  VLFc=1  angleLF=0  angleLFb=0  angleLFc=0
      settings: SourceProductBaseCode=PS
  Neutral{,1..20} (21 alike) : spsNeutralLib/Neutral  LConnTagsString=a  NodeNumber=10
      settings: AttributesFormatString=node %<NodeNumber>  SourceProductBaseCode=PS
  RELIGADOR : Subsystem
  RELIGADOR1 : Subsystem
  RMS{5..24} (20 alike) : dspstat3/RMS  run=on  directionMode=Each column  dimension=1  InputProcessing=Columns as channels (frame based)  reset_popup=None
  Relé Sobrecorrente : Subsystem
  Relé Sobrecorrente1 : Subsystem
  SUB : spsThreePhaseSourceLib/Three-Phase Source  InternalConnection=Yn  VoltagePhases=off  Voltage=(69e3)*1.05  PhaseAngle=30  Voltage_phases=[69e3 69e3 69e3]/sqrt(3)  PhaseAngles_phases=[0 -120 +120]  Frequency=60  NonIdealSource=on  SpecifyImpedance=on  Resistance=0.8929  Inductance=16.58e-3  ShortCircuitLevel=200000e6  BaseVoltage=69e3  XRratio=7  BusType=swing  Pref=10e3  Qref=0  Prefabc=[10e3, 10e3, 10e3]  Qrefabc=[0, 0, 0]  Qmin=-inf  Qmax=inf
  Scope : Scope  NumInputPorts=3
  Scope1 : Scope  NumInputPorts=2
  Scope3 : Scope  NumInputPorts=2
  Scope6 : Scope  Commented=on  NumInputPorts=3
  Sum{2..6} (5 alike) : Sum  Inputs=3
  TSUB : spsThreePhaseTransformerTwoWindingsLib/Three-Phase Transformer (Two Windings)  Winding1Connection=Delta (D1)  Winding2Connection=Yg  CoreType=Three single-phase transformers  SetSaturation=off  Hysteresis=off  DataFile='hysteresis'  SetInitialFlux=off  Measurements=None  UNITS=pu  NominalPower=[ 2500e3 , 60 ]  Winding1=[ 69e3 , 0.001 , 0.1001 ]  Winding2=[ 24.9e3 , 0.001 , 0.1001 ]  Rm=500  Lm=500  L0=0.5  Saturation=[ 0,0 ; 0.0024,1.2 ; 1.0,1.52 ]  InitialFluxes=[ 0.8 , -0.8 , 0.7 ]  BreakLoop=off  DiscreteSolver=Trapezoidal iterative  DataType=off  TransfoNumber=1
  Three-Phase Breaker1 : spsThreePhaseBreakerLib/Three-Phase Breaker  InitialState=closed  SwitchA=on  SwitchB=on  SwitchC=on  SwitchTimes=5.0  External=on  BreakerResistance=0.01  SnubberResistance=1e6  SnubberCapacitance=inf  Measurements=None
  Three-Phase Breaker2 : spsThreePhaseBreakerLib/Three-Phase Breaker  InitialState=closed  SwitchA=on  SwitchB=on  SwitchC=on  SwitchTimes=5.0  External=on  BreakerResistance=0.01  SnubberResistance=1e6  SnubberCapacitance=inf  Measurements=None
  Three-Phase Breaker3 : spsThreePhaseBreakerLib/Three-Phase Breaker  InitialState=closed  SwitchA=on  SwitchB=on  SwitchC=on  SwitchTimes=5.0  External=off  BreakerResistance=0.01  SnubberResistance=1e6  SnubberCapacitance=inf  Measurements=None
  Three-Phase Breaker4 : spsThreePhaseBreakerLib/Three-Phase Breaker  InitialState=closed  SwitchA=on  SwitchB=off  SwitchC=off  SwitchTimes=5.0  External=on  BreakerResistance=0.01  SnubberResistance=1e6  SnubberCapacitance=inf  Measurements=None
  Three-Phase Breaker5 : spsThreePhaseBreakerLib/Three-Phase Breaker  Commented=on  InitialState=closed  SwitchA=on  SwitchB=on  SwitchC=on  SwitchTimes=5.0  External=on  BreakerResistance=0.01  SnubberResistance=1e6  SnubberCapacitance=inf  Measurements=None
  Three-Phase Fault1 : spsThreePhaseFaultLib/Three-Phase Fault  Commented=on  InitialStates=0  FaultA=on  FaultB=on  FaultC=on  GroundFault=off  SwitchTimes=[0.2 2]  External=off  SwitchStatus=NaN  FaultResistance=0.001  GroundResistance=0.01  SnubberResistance=1e6  SnubberCapacitance=inf  Measurements=None
  Three-Phase Fault2 : spsThreePhaseFaultLib/Three-Phase Fault  Commented=on  InitialStates=0  FaultA=off  FaultB=on  FaultC=off  GroundFault=on  SwitchTimes=0.3  External=off  SwitchStatus=NaN  FaultResistance=0.001  GroundResistance=0.01  SnubberResistance=1e6  SnubberCapacitance=inf  Measurements=None
  Three-Phase Fault3 : spsThreePhaseFaultLib/Three-Phase Fault  Commented=on  InitialStates=0  FaultA=on  FaultB=off  FaultC=off  GroundFault=on  SwitchTimes=[0.2 3]  External=off  SwitchStatus=NaN  FaultResistance=0.001  GroundResistance=0.01  SnubberResistance=1e6  SnubberCapacitance=inf  Measurements=None
  Three-Phase Fault4 : spsThreePhaseFaultLib/Three-Phase Fault  Commented=on  InitialStates=0  FaultA=on  FaultB=off  FaultC=on  GroundFault=on  SwitchTimes=0.2  External=off  SwitchStatus=NaN  FaultResistance=0.001  GroundResistance=0.01  SnubberResistance=1e6  SnubberCapacitance=inf  Measurements=None
  Three-Phase Fault5 : spsThreePhaseFaultLib/Three-Phase Fault  InitialStates=0  FaultA=on  FaultB=off  FaultC=off  GroundFault=on  SwitchTimes=0.3  External=off  SwitchStatus=NaN  FaultResistance=0.001  GroundResistance=0.01  SnubberResistance=1e6  SnubberCapacitance=inf  Measurements=None
  Three-Phase Fault6 : spsThreePhaseFaultLib/Three-Phase Fault  Commented=on  InitialStates=0  FaultA=off  FaultB=on  FaultC=on  GroundFault=off  SwitchTimes=[0.2 2]  External=off  SwitchStatus=NaN  FaultResistance=0.001  GroundResistance=0.01  SnubberResistance=1e6  SnubberCapacitance=inf  Measurements=None
  Three-Phase Fault7 : spsThreePhaseFaultLib/Three-Phase Fault  Commented=on  InitialStates=0  FaultA=on  FaultB=on  FaultC=on  GroundFault=on  SwitchTimes=[0.2 1]  External=off  SwitchStatus=NaN  FaultResistance=0.001  GroundResistance=0.01  SnubberResistance=1e6  SnubberCapacitance=inf  Measurements=None
  To Workspace11 : ToWorkspace  Commented=on  VariableName=corrente_832  SaveFormat=Timeseries  SampleTime=-1
  To Workspace12 : ToWorkspace  Commented=on  VariableName=trip_832  SaveFormat=Timeseries  SampleTime=-1
  To Workspace2 : ToWorkspace  VariableName=Out_800  SampleTime=-1
      settings: Save2DSignal=2-D array (concatenate along first dimension)
  To Workspace3 : ToWorkspace  VariableName=Out_832  SampleTime=-1
      settings: Save2DSignal=2-D array (concatenate along first dimension)
  To Workspace4 : ToWorkspace  VariableName=Out_834  SampleTime=-1
      settings: Save2DSignal=2-D array (concatenate along first dimension)
  To Workspace5 : ToWorkspace  VariableName=Out_836  SampleTime=-1
      settings: Save2DSignal=2-D array (concatenate along first dimension)
  To Workspace6 : ToWorkspace  VariableName=Out_842  SampleTime=-1
      settings: Save2DSignal=2-D array (concatenate along first dimension)
  XFM-1 : spsThreePhaseTransformerTwoWindingsLib/Three-Phase Transformer (Two Windings)  Winding1Connection=Yg  Winding2Connection=Yg  CoreType=Three single-phase transformers  SetSaturation=off  Hysteresis=off  DataFile='hysteresis'  SetInitialFlux=off  Measurements=None  UNITS=pu  NominalPower=[ 500e3 , 60 ]  Winding1=[ 24.9e3 , 0.019 , 0.0408 ]  Winding2=[ 4.16e3 , 0.019 , 0.0408 ]  Rm=500  Lm=500  L0=0.5  Saturation=[ 0,0 ; 0.0024,1.2 ; 1.0,1.52 ]  InitialFluxes=[ 0.8 , -0.8 , 0.7 ]  BreakLoop=off  DiscreteSolver=Trapezoidal iterative  DataType=off  TransfoNumber=1
  powergui : spspowerguiLib/powergui  Priority=1  SimulationMode=Discrete  SampleTime=5e-5  frequency=60  Iterations=50  frequencyindice=0  Pbase=100e6  ErrMax=1e-4  UnitsV=kV  UnitsW=MW  buscounter=0  FunctionMessages=off  echomessages=off  EnableUseOfTLC=off  CurrentSourceSwitches=off  DisableSnubberDevices=off  DisableRonSwitches=off  DisableVfSwitches=off  DisplayEquations=off  AutomaticDiscreteSolvers=off  SolverType=Tustin/Backward Euler (TBE)  Interpol=off  ExternalGateDelay=off  methode=off  Ts=0  x0status=blocks  SPID=off  SwTol=0  HookPort=off  NonlinearTolerance=1e-8  nMaxIteration=10  ContinueOnMaxIteration=off  RestoreLinks=warning  ResistiveCurrentMeasurement=off  Frange=[0:2:500]  Ylog=off  Xlog=on  ShowGrid=off  save=off  variable=ZData  structure=0  ZoomFFT=on  StartTime=0.0  cycles=1  DisplayStyle=1  fundamental=60  FreqAxis=off  MaxFrequency=1000  frequencyindicesteady=1  RmsSteady=1  display=off
  wires:
  [Trip800] -> Three-Phase Breaker1/1
  Bus Creator3/1 -> To Workspace3/1
  [Ic834] -> Bus Creator4/7
  RMS13/1 -> Ib4/1
  RMS16/1 -> Ia4/1
  [Va834] -> Bus Creator4/2
  [Ic832] -> Bus Creator3/7
  [Ia800] -> Sum2/1
  Relé Sobrecorrente/2(Out2) -> [Trp800]
  Demux8/3 -> [Vc834]
  Demux7/1 -> [Ia834]
  [Ib834] -> Bus Creator4/6
  RMS7/1 -> Ib_1/1
  Demux7/2 -> [Ib834]
  [Ib834] -> Sum4/2
  Sum3/1 -> RMS5/1
  [t] -> Bus Creator4/1
  [Vb832] -> Bus Creator3/3
  [Va800] -> Bus Creator1/2
  [Ia832] -> RMS9/1
  [Vb800] -> Relé Sobrecorrente/2(In2)
  [Iabc_834] -> Demux7/1
  Demux2/1 -> [Ia800]
  [Trp832] -> Bus Creator3/8
  Sum4/1 -> RMS15/1
  [Trp800] -> Bus Creator1/8
  [Vc800] -> Bus Creator1/4
  [Ia834] -> RMS16/1
  [Ic834] -> RMS14/1
  RMS14/1 -> Ic4/1
  Demux7/3 -> [Ic834]
  Demux8/2 -> [Vb834]
  RMS15/1 -> "In4 "/1
  Bus Creator4/1 -> To Workspace4/1
  [Ib834] -> RMS13/1
  [Ic800] -> RMS8/1
  [Ia832] -> Bus Creator3/5
  [Vabc_834] -> Demux8/1
  [Ic834] -> Sum4/3
  [Vb800] -> Bus Creator1/3
  [Ic832] -> RMS12/1
  [Va800] -> Relé Sobrecorrente/1(In1)  "Va"
  Relé Sobrecorrente/1(Out1) -> [Trip800]
  [t] -> Bus Creator3/1
  [Vc800] -> Relé Sobrecorrente/3(In3)
  [Ia834] -> Sum4/1
  [Vc832] -> Bus Creator3/4
  [Ib832] -> Bus Creator3/6
  Demux5/1 -> [Ia832]
  [Ia834] -> Bus Creator4/5
  Bus Creator1/1 -> To Workspace2/1
  [Vabc_832] -> Demux6/1
  [Ib800] -> Relé Sobrecorrente/5(In5)
  [Ia832] -> Sum3/1
  [Ib832] -> RMS10/1
  RMS9/1 -> Ia3/1
  Demux2/2 -> [Ib800]
  Demux3/1 -> [Va800]
  Demux5/3 -> [Ic832]
  [Iabc_832] -> Demux5/1
  Demux8/1 -> [Va834]
  Demux5/2 -> [Ib832]
  [Vabc_800] -> Demux3/1
  [Vb834] -> Bus Creator4/3
  Demux6/2 -> [Vb832]
  [Ia800] -> Relé Sobrecorrente/4(In4)
  Demux6/3 -> [Vc832]
  RMS10/1 -> Ib3/1
  [Ib800] -> RMS7/1
  [Ic800] -> Relé Sobrecorrente/6(In6)
  [Vc834] -> Bus Creator4/4
  RMS8/1 -> Ic_1/1
  Sum2/1 -> RMS11/1
  Demux6/1 -> [Va832]
  RMS11/1 -> "In_1 "/1
  [Ib832] -> Sum3/2
  [Ic800] -> Sum2/3
  [Ib800] -> Sum2/2
  [Ic832] -> Sum3/3
  [Va832] -> Bus Creator3/2
  RMS5/1 -> "In3 "/1
  [Ia800] -> RMS6/1
  [Ic800] -> Bus Creator1/7
  [Ib800] -> Bus Creator1/6
  [t] -> Bus Creator1/1
  Demux3/3 -> [Vc800]
  RMS12/1 -> Ic3/1
  Demux2/3 -> [Ic800]
  [Ia800] -> Bus Creator1/5
  [Iabc_800] -> Demux2/1
  Clock1/1 -> [t]
  Demux3/2 -> [Vb800]
  RMS6/1 -> Ia_1/1
  From45/1 -> Three-Phase Breaker5/1
  [Vc836] -> Bus Creator5/4
  Demux10/1 -> [Va836]
  [Ia836] -> Bus Creator5/5
  [Vabc_836] -> Demux10/1
  [Ib836] -> RMS17/1
  Bus Creator5/1 -> To Workspace5/1
  [Ia836] -> Sum5/1
  RMS19/1 -> In4 1/1
  [Ic836] -> RMS18/1
  Sum5/1 -> RMS19/1
  [Iabc_836] -> Demux9/1
  [t] -> Bus Creator5/1
  [Ia836] -> RMS20/1
  [Ic836] -> Sum5/3
  [Ib836] -> Bus Creator5/6
  [Ib836] -> Sum5/2
  Demux9/1 -> [Ia836]
  [Va836] -> Bus Creator5/2
  Demux10/3 -> [Vc836]
  RMS17/1 -> Ib1/1
  Demux9/2 -> [Ib836]
  [Ic836] -> Bus Creator5/7
  Demux9/3 -> [Ic836]
  RMS20/1 -> Ia1/1
  Demux10/2 -> [Vb836]
  RMS18/1 -> Ic1/1
  [Vb836] -> Bus Creator5/3
  [Trp836] -> Bus Creator5/8
  Demux11/3 -> [Vc842]
  [Iabc_842] -> Demux12/1
  RMS22/1 -> Ic5/1
  Demux12/2 -> [Ib842]
  [Ia842] -> Bus Creator6/5
  Demux12/3 -> [Ic842]
  [Ib842] -> Sum6/2
  [Va842] -> Bus Creator6/2
  Demux11/1 -> [Va842]
  [Vb842] -> Bus Creator6/3
  [Ib842] -> RMS21/1
  [Ia842] -> RMS24/1
  RMS24/1 -> Ia5/1
  [Ib842] -> Bus Creator6/6
  Bus Creator6/1 -> To Workspace6/1
  [Ic842] -> Sum6/3
  [t] -> Bus Creator6/1
  [Ia842] -> Sum6/1
  [Vc842] -> Bus Creator6/4
  [Ic842] -> RMS22/1
  RMS23/1 -> In4 2/1
  Demux12/1 -> [Ia842]
  Sum6/1 -> RMS23/1
  [Vabc_842] -> Demux11/1
  [Trp842] -> Bus Creator6/8
  [Ic842] -> Bus Creator6/7
  Demux11/2 -> [Vb842]
  RMS21/1 -> Ib5/1
  [Vabc_800] -> Scope/1
  [Iabc_800] -> Scope/2
  [Trp800] -> Scope/3
  From180/1 -> Scope6/2, To Workspace11/1
  From179/1 -> Scope6/1
  From181/1 -> To Workspace12/1, Scope6/3
  [Trp834] -> Bus Creator4/8
  [Ia834] -> RELIGADOR/4(In4)
  [Vc834] -> RELIGADOR/3(In3)
  [Ic834] -> RELIGADOR/6(In6)
  [Vb834] -> RELIGADOR/2(In2)
  [Va834] -> RELIGADOR/1(In1)  "Va"
  [Ib834] -> RELIGADOR/5(In5)
  [teste] -> Three-Phase Breaker2/1
  RELIGADOR/1(Out1) -> [teste]
  RELIGADOR/2(Out3) -> [trip_teste]
  RELIGADOR1/2(Out3) -> [trip_teste1]
  RELIGADOR1/1(Out1) -> [teste1]
  [Ia_3_2] -> RELIGADOR1/4(In4)
  [Va_3_2] -> RELIGADOR1/1(In1)  "Va"
  [Vb_3_2] -> RELIGADOR1/2(In2)
  [Ib_3_2] -> RELIGADOR1/5(In5)
  [Vc_3_2] -> RELIGADOR1/3(In3)
  [Ic_3_2] -> RELIGADOR1/6(In6)
  [teste1] -> ?
  Demux1/3 -> [Ic824]
  Demux1/2 -> [Ib824]
  [Iabc_824] -> Demux1/1
  Demux1/1 -> [Ia824]
  Demux4/3 -> [Vc824]
  Demux4/2 -> [Vb824]
  [Vabc_824] -> Demux4/1
  Demux4/1 -> [Va824]
  [Trip_F1] -> Three-Phase Breaker4/1
  Demux13/3 -> [Ic_3_2]
  Demux14/3 -> [Vc_3_2]
  Demux13/2 -> [Ib_3_2]
  Demux14/2 -> [Vb_3_2]
  Demux14/1 -> [Va_3_2]
  [Iabc_3_2] -> Demux13/1
  Demux13/1 -> [Ia_3_2]
  [Vabc_3_2] -> Demux14/1
  [Ia800] -> Relé Sobrecorrente1/4(In4)
  [Va800] -> Relé Sobrecorrente1/1(In1)  "Va"
  [Ib800] -> Relé Sobrecorrente1/5(In5)
  [Vc800] -> Relé Sobrecorrente1/3(In3)
  [Vb800] -> Relé Sobrecorrente1/2(In2)
  [Ic800] -> Relé Sobrecorrente1/6(In6)
  Relé Sobrecorrente1/1(Out3) -> [Trip_F1]
  [Iabc_824] -> Scope3/1
  [trip_teste1] -> Scope3/2
  [Iabc_834] -> Scope1/1
  [trip_teste] -> Scope1/2
  connections:
  BSUB/RConn1 -- SUB/RConn3
  BSUB/RConn2 -- SUB/RConn2
  BSUB/RConn3 -- SUB/RConn1
  TSUB/RConn1 -- 800/RConn3
  TSUB/RConn2 -- 800/RConn2
  TSUB/RConn3 -- 800/RConn1
  812/RConn3 -- L808-812 config 300/RConn1
  812/RConn2 -- L808-812 config 300/RConn2
  812/RConn1 -- L808-812 config 300/RConn3
  L812-814 config 300/LConn1 -- Three-Phase Fault1/LConn1 -- 812/LConn3
  L812-814 config 300/LConn2 -- Three-Phase Fault1/LConn2 -- 812/LConn2
  L812-814 config 300/LConn3 -- Three-Phase Fault1/LConn3 -- 812/LConn1
  814/RConn1 -- L812-814 config 300/RConn3
  814/RConn2 -- L812-814 config 300/RConn2
  814/RConn3 -- L812-814 config 300/RConn1
  L802-806b config 300/LConn1 -- L802-806a config 300/RConn1
  L802-806b config 300/LConn2 -- 802-806 b Y-PQ/LConn1 -- L802-806a config 300/RConn2
  L802-806b config 300/LConn3 -- 802-806 c Y-PQ/LConn1 -- L802-806a config 300/RConn3
  L802-806b config 300/RConn3 -- 806/RConn1
  L802-806b config 300/RConn2 -- 806/RConn2
  L802-806b config 300/RConn1 -- 806/RConn3
  " L808-810a config 303 "/RConn1 -- Load 808-810 Y-I/LConn1 -- " L808-810b config 303 "/LConn1
  Load Flow Bus/LConn1 -- " L808-810b config 303 "/RConn1
  Neutral3/LConn1 -- Load 808-810 Y-I/RConn1
  Neutral2/LConn1 -- 802-806 b Y-PQ/RConn1
  Neutral1/LConn1 -- 802-806 c Y-PQ/RConn1
  L814-850 config 301/LConn1 -- 814/LConn3
  L814-850 config 301/LConn2 -- 814/LConn2
  L814-850 config 301/LConn3 -- 814/LConn1
  850/RConn1 -- L814-850 config 301/RConn3
  850/RConn2 -- L814-850 config 301/RConn2
  850/RConn3 -- L814-850 config 301/RConn1
  L850-816 config 301/LConn1 -- 850/LConn3
  L850-816 config 301/LConn2 -- 850/LConn2
  L850-816 config 301/LConn3 -- 850/LConn1
  " L818-820a config 302"/LConn1 -- " L816-818 config 302"/RConn1
  " L818-820b config 302"/LConn1 -- 818-820 Y-Z/LConn1 -- " L818-820a config 302"/RConn1
  Neutral5/LConn1 -- 818-820 Y-Z/RConn1
  " L820-822a config 302"/LConn1 -- " L818-820b config 302"/RConn1
  " L820-822b config 302"/LConn1 -- 820-822 Y-PQ/LConn1 -- " L820-822a config 302"/RConn1
  Neutral4/LConn1 -- 820-822 Y-PQ/RConn1
  " L824-826b config 303 "/RConn1 -- " 824-826 Y-I"/LConn1 -- " L824-826a config 303 "/LConn1
  Neutral6/LConn1 -- " 824-826 Y-I"/RConn1
  L828-830a config 301/LConn1 -- 828/LConn3
  L828-830a config 301/LConn2 -- 828/LConn2
  L828-830a config 301/LConn3 -- 828/LConn1
  L824-828b config 301/LConn1 -- L824-828a config 301/RConn1
  L824-828b config 301/LConn2 -- L824-828a config 301/RConn2
  L824-828b config 301/LConn3 -- L824-828a config 301/RConn3 -- Load 824-828 Y-PQ/LConn1
  L824-828b config 301/RConn1 -- 828/RConn3
  828/RConn2 -- L824-828b config 301/RConn2
  L824-828b config 301/RConn3 -- 828/RConn1
  Neutral7/LConn1 -- Load 824-828 Y-PQ/RConn1
  L816-824b config 301/LConn1 -- L816-824a config 301/RConn1
  L816-824b config 301/LConn2 -- " 816-824 D-I"/LConn1 -- L816-824a config 301/RConn2
  L816-824b config 301/LConn3 -- L816-824a config 301/RConn3 -- " 816-824 D-I"/RConn1
  L828-830b config 301/LConn1 -- " 828-830 Y-PQ"/LConn1 -- L828-830a config 301/RConn1
  L828-830b config 301/LConn2 -- L828-830a config 301/RConn2
  L828-830b config 301/LConn3 -- L828-830a config 301/RConn3
  " L854-856a config 303 "/LConn1 -- " 854-856 Y-PQ"/LConn1 -- " L854-856b config 303 "/RConn1
  852/RConn3 -- L854-852 config 301/RConn1
  852/RConn2 -- L854-852 config 301/RConn2
  852/RConn1 -- L854-852 config 301/RConn3
  L852-832 config 301/LConn1 -- 852/LConn3
  L852-832 config 301/LConn2 -- 852/LConn2
  L852-832 config 301/LConn3 -- 852/LConn1
  888/RConn3 -- XFM-1/RConn1
  888/RConn2 -- XFM-1/RConn2
  888/RConn1 -- XFM-1/RConn3
  L888-890 config 300/LConn1 -- 888/LConn3
  L888-890 config 300/LConn2 -- 888/LConn2
  L888-890 config 300/LConn3 -- 888/LConn1
  890/RConn3 -- L888-890 config 300/RConn1
  890/RConn2 -- L888-890 config 300/RConn2
  890/RConn1 -- L888-890 config 300/RConn3
  " Load 890 D-I"/LConn1 -- 890/LConn3
  " Load 890 D-I"/LConn2 -- 890/LConn2
  " Load 890 D-I"/LConn3 -- 890/LConn1
  L832-858b config 301/LConn1 -- 832-858 D-Z/RConn1 -- 832-858a D-Z/LConn1 -- L832-858a config 301/RConn1 -- Three-Phase Fault7/LConn1
  L832-858b config 301/LConn2 -- 832-858b D-Z/LConn1 -- 832-858a D-Z/RConn1 -- Three-Phase Fault7/LConn2 -- L832-858a config 301/RConn2
  L832-858b config 301/LConn3 -- 832-858 D-Z/LConn1 -- 832-858b D-Z/RConn1 -- Three-Phase Fault7/LConn3 -- L832-858a config 301/RConn3
  L858-834b config 301/LConn1 -- 858-834a D-PQ/LConn1 -- L858-834a config 301/RConn1 -- 858-834c D-PQ/RConn1
  L858-834b config 301/LConn2 -- 858-834b D-PQ/LConn1 -- 858-834a D-PQ/RConn1 -- L858-834a config 301/RConn2
  L858-834b config 301/LConn3 -- 858-834c D-PQ/LConn1 -- 858-834b D-PQ/RConn1 -- L858-834a config 301/RConn3
  " L858-864b config 302"/LConn1 -- 858-864 Y-PQ/LConn1 -- " L858-864a config 302"/RConn1
  842/RConn3 -- L834-842 config 301/RConn1
  842/RConn2 -- L834-842 config 301/RConn2
  842/RConn1 -- L834-842 config 301/RConn3
  L842-844b config 301/LConn1 -- L842-844a config 301/RConn1 -- 842-844 Y-PQ/LConn1
  L842-844b config 301/LConn2 -- L842-844a config 301/RConn2
  L842-844b config 301/LConn3 -- L842-844a config 301/RConn3
  844/RConn4 -- L842-844b config 301/RConn1
  844/RConn5 -- L842-844b config 301/RConn2
  844/RConn6 -- L842-844b config 301/RConn3
  L844-846a config 301/LConn1 -- 844/LConn4
  L844-846a config 301/LConn2 -- 844/LConn5
  L844-846a config 301/LConn3 -- 844/LConn6
  L844-846b config 301/LConn1 -- L844-846a config 301/RConn1 -- Three-Phase Fault6/LConn1
  L844-846b config 301/LConn2 -- Three-Phase Fault6/LConn2 -- 844-846b Y-PQ/LConn1 -- L844-846a config 301/RConn2
  L844-846b config 301/LConn3 -- 844-846c Y-PQ2/LConn1 -- Three-Phase Fault6/LConn3 -- L844-846a config 301/RConn3
  846/RConn1 -- L844-846b config 301/RConn3
  846/RConn2 -- L844-846b config 301/RConn2
  846/RConn3 -- L844-846b config 301/RConn1
  L846-848a config 301/LConn1 -- 846/LConn3
  L846-848a config 301/LConn2 -- 846/LConn2
  L846-848a config 301/LConn3 -- 846/LConn1
  L846-848b config 301/LConn1 -- L846-848a config 301/RConn1
  L846-848b config 301/LConn2 -- 846-848b Y-PQ/LConn1 -- L846-848a config 301/RConn2
  L846-848b config 301/LConn3 -- L846-848a config 301/RConn3
  " Load 844 Y-Z"/LConn1 -- 844/LConn7
  " Load 844 Y-Z"/LConn2 -- 844/LConn8
  " Load 844 Y-Z"/LConn3 -- 844/LConn9
  L834-860b config 301/LConn1 -- 834-860a D-Z/LConn1 -- L834-860a config 301/RConn1 -- 834-860c D-Z/RConn1
  L834-860b config 301/LConn2 -- 834-860b D-Z/LConn1 -- 834-860a D-Z/RConn1 -- L834-860a config 301/RConn2
  L834-860b config 301/LConn3 -- 834-860c D-Z/LConn1 -- 834-860b D-Z/RConn1 -- L834-860a config 301/RConn3
  860/LConn4 -- L834-860b config 301/RConn1
  860/LConn5 -- L834-860b config 301/RConn2
  860/LConn6 -- L834-860b config 301/RConn3
  " Load 860 Y-PQ"/LConn1 -- 860/LConn7
  " Load 860 Y-PQ"/LConn2 -- 860/LConn8
  " Load 860 Y-PQ"/LConn3 -- 860/LConn9
  L860-836a config 301/LConn1 -- Three-Phase Fault2/LConn1 -- 860/RConn4
  L860-836a config 301/LConn2 -- Three-Phase Fault2/LConn2 -- 860/RConn5
  L860-836a config 301/LConn3 -- Three-Phase Fault2/LConn3 -- 860/RConn6
  L860-836b config 301/LConn1 -- L860-836a config 301/RConn1 -- 860-836a D-PQ/LConn1 -- 860-836c D-PQ/RConn1
  L860-836b config 301/LConn2 -- 860-836a D-PQ/RConn1 -- L860-836a config 301/RConn2 -- 860-836b D-PQ/LConn1
  L860-836b config 301/LConn3 -- 860-836b D-PQ/RConn1 -- L860-836a config 301/RConn3 -- 860-836c D-PQ/LConn1
  L836-840b config 301/LConn1 -- 836-840a D-I/LConn1 -- L836-840a config 301/RConn1
  L836-840b config 301/LConn2 -- 836-840b D-I/LConn1 -- 836-840a D-I/RConn1 -- L836-840a config 301/RConn2
  L836-840b config 301/LConn3 -- 836-840b D-I/RConn1 -- L836-840a config 301/RConn3
  840/RConn3 -- L836-840b config 301/RConn1
  840/RConn1 -- L836-840b config 301/RConn3
  840/RConn2 -- L836-840b config 301/RConn2
  862/LConn3 -- L836-862 config 301/RConn1
  862/LConn2 -- L836-862 config 301/RConn2
  862/LConn1 -- L836-862 config 301/RConn3
  " L862-838a config 304"/RConn1 -- 862/RConn2
  " L862-838b config 304"/RConn1 -- 862-838 Y-PQ/LConn1 -- " L862-838a config 304"/LConn1
  Capacitor 844/LConn1 -- 844/LConn1
  Capacitor 844/LConn2 -- 844/LConn2
  Capacitor 844/LConn3 -- 844/LConn3
  848/LConn4 -- " Load 848 D-PQ"/LConn1
  848/LConn5 -- " Load 848 D-PQ"/LConn2
  848/LConn6 -- " Load 848 D-PQ"/LConn3
  848/RConn4 -- L846-848b config 301/RConn1
  848/RConn5 -- L846-848b config 301/RConn2
  848/RConn6 -- L846-848b config 301/RConn3
  Capacitor 848/LConn1 -- 848/LConn7
  Capacitor 848/LConn2 -- 848/LConn8
  Capacitor 848/LConn3 -- 848/LConn9
  808/LConn4 -- L806-808 config 300/RConn1
  808/LConn5 -- L806-808 config 300/RConn2
  808/LConn6 -- L806-808 config 300/RConn3
  Load Flow Bar1/LConn1 -- 800/LConn3
  Load Flow Bar1/LConn2 -- 800/LConn2
  Load Flow Bar1/LConn3 -- 800/LConn1
  Load Flow Bar2/RConn1 -- L802-806a config 300/LConn1
  L802-806a config 300/LConn2 -- Load Flow Bar2/RConn2
  L802-806a config 300/LConn3 -- Load Flow Bar2/RConn3
  Load Flow Bar/LConn1 -- BSUB/LConn3
  Load Flow Bar/LConn2 -- BSUB/LConn2
  BSUB/LConn1 -- Load Flow Bar/LConn3
  Load Flow Bar/RConn1 -- TSUB/LConn1
  TSUB/LConn2 -- Load Flow Bar/RConn2
  Load Flow Bar/RConn3 -- TSUB/LConn3
  Load Flow Bar2/LConn1 -- L800-802 config 300/RConn1
  Load Flow Bar2/LConn2 -- L800-802 config 300/RConn2
  Load Flow Bar2/LConn3 -- L800-802 config 300/RConn3
  Load Flow Bar3/RConn1 -- L806-808 config 300/LConn1
  Load Flow Bar3/RConn2 -- L806-808 config 300/LConn2
  Load Flow Bar3/RConn3 -- L806-808 config 300/LConn3
  Load Flow Bar3/LConn1 -- 806/LConn3
  Load Flow Bar3/LConn2 -- 806/LConn2
  Load Flow Bar3/LConn3 -- 806/LConn1
  Load Flow Bar4/LConn1 -- 808/RConn4
  Load Flow Bar4/LConn2 -- Three-Phase Breaker4/RConn2 -- 808/RConn5
  Load Flow Bar4/LConn3 -- 808/RConn6
  Load Flow Bar4/RConn1 -- L808-812 config 300/LConn1
  Load Flow Bar4/RConn2 -- L808-812 config 300/LConn2
  Load Flow Bar4/RConn3 -- L808-812 config 300/LConn3
  Neutral/LConn1 -- SUB/LConn1
  Neutral8/LConn1 -- " 828-830 Y-PQ"/RConn1
  Neutral9/LConn1 -- " 854-856 Y-PQ"/RConn1
  Neutral10/LConn1 -- 858-864 Y-PQ/RConn1
  Neutral11/LConn1 -- 842-844 Y-PQ/RConn1
  Neutral12/LConn1 -- 844-846b Y-PQ/RConn1
  Neutral14/LConn1 -- 846-848b Y-PQ/RConn1
  Neutral17/LConn1 -- " Load 860 Y-PQ"/RConn1
  Neutral18/LConn1 -- " Load 840 Y-I"/RConn1
  Neutral19/LConn1 -- 862-838 Y-PQ/RConn1
  Neutral20/LConn1 -- " Load 844 Y-Z"/RConn1
  Neutral15/LConn1 -- Capacitor 844/RConn1
  Neutral16/LConn1 -- Capacitor 848/RConn1
  Load Flow Bus1/LConn1 -- " L820-822b config 302"/RConn1
  Load Flow Bus2/LConn1 -- " L824-826b config 303 "/LConn1
  Load Flow Bus3/LConn1 -- " L854-856b config 303 "/LConn1
  Neutral13/LConn1 -- 844-846c Y-PQ2/RConn1
  816/LConn3 -- L816-824a config 301/LConn1 -- " L816-818 config 302"/LConn1
  816/RConn3 -- L850-816 config 301/RConn1
  816/RConn2 -- L850-816 config 301/RConn2
  816/RConn1 -- L850-816 config 301/RConn3
  824/RConn3 -- L816-824b config 301/RConn1
  824/RConn2 -- L816-824b config 301/RConn2
  824/RConn1 -- L816-824b config 301/RConn3
  " L824-826a config 303 "/RConn1 -- Three-Phase Breaker3/RConn2 -- 824/LConn2
  830/RConn3 -- L828-830b config 301/RConn1
  830/LConn3 -- Three-Phase Fault3/LConn1 -- L830-854 config 301/LConn1 -- " Load 830 D-Z"/LConn1
  830/LConn2 -- Three-Phase Fault3/LConn2 -- L830-854 config 301/LConn2 -- " Load 830 D-Z"/LConn2
  830/RConn2 -- L828-830b config 301/RConn2
  830/RConn1 -- L828-830b config 301/RConn3
  830/LConn1 -- Three-Phase Fault3/LConn3 -- L830-854 config 301/LConn3 -- " Load 830 D-Z"/LConn3
  854/RConn3 -- L830-854 config 301/RConn1
  854/RConn2 -- L830-854 config 301/RConn2
  854/RConn1 -- L830-854 config 301/RConn3
  854/LConn2 -- Three-Phase Fault4/LConn2 -- L854-852 config 301/LConn2 -- " L854-856a config 303 "/RConn1
  854/LConn3 -- Three-Phase Fault4/LConn1 -- L854-852 config 301/LConn1
  L854-852 config 301/LConn3 -- Three-Phase Fault4/LConn3 -- 854/LConn1
  832/RConn1 -- L852-832 config 301/RConn3
  832/RConn2 -- L852-832 config 301/RConn2
  832/RConn3 -- L852-832 config 301/RConn1
  858/RConn3 -- L832-858b config 301/RConn1
  858/RConn2 -- L832-858b config 301/RConn2
  858/RConn1 -- L832-858b config 301/RConn3
  858/LConn3 -- L858-834a config 301/LConn1 -- " L858-864a config 302"/LConn1
  L858-834a config 301/LConn2 -- 858/LConn2
  L858-834a config 301/LConn3 -- 858/LConn1
  834/RConn3 -- L858-834b config 301/RConn1
  834/RConn2 -- L858-834b config 301/RConn2
  Three-Phase Breaker2/LConn3 -- 834/LConn1
  L858-834b config 301/RConn3 -- 834/RConn1
  832/LConn3 -- XFM-1/LConn1 -- L832-858a config 301/LConn1
  832/LConn2 -- XFM-1/LConn2 -- L832-858a config 301/LConn2
  832/LConn1 -- L832-858a config 301/LConn3 -- XFM-1/LConn3
  842/LConn1 -- Three-Phase Fault5/LConn3 -- L842-844a config 301/LConn3
  842/LConn2 -- Three-Phase Fault5/LConn2 -- L842-844a config 301/LConn2
  842/LConn3 -- Three-Phase Fault5/LConn1 -- L842-844a config 301/LConn1
  836/RConn3 -- L860-836b config 301/RConn1
  836/RConn2 -- L860-836b config 301/RConn2
  836/RConn1 -- L860-836b config 301/RConn3
  L836-862 config 301/LConn3 -- L836-840a config 301/LConn3 -- 836/LConn1
  L836-862 config 301/LConn1 -- L836-840a config 301/LConn1 -- 836/LConn3
  L836-862 config 301/LConn2 -- L836-840a config 301/LConn2 -- 836/LConn2
  " Load 840 Y-I"/LConn1 -- 840/LConn3
  " Load 840 Y-I"/LConn3 -- 840/LConn1
  " Load 840 Y-I"/LConn2 -- 840/LConn2
  L816-824a config 301/LConn2 -- 816/LConn2
  L816-824a config 301/LConn3 -- 816/LConn1
  Three-Phase Breaker2/LConn1 -- 834/LConn3
  Three-Phase Breaker2/LConn2 -- 834/LConn2
  Three-Phase Breaker2/RConn1 -- L834-842 config 301/LConn1 -- L834-860a config 301/LConn1
  Three-Phase Breaker2/RConn2 -- L834-842 config 301/LConn2 -- L834-860a config 301/LConn2
  Three-Phase Breaker2/RConn3 -- L834-842 config 301/LConn3 -- L834-860a config 301/LConn3
  L824-828a config 301/LConn1 -- Three-Phase Breaker3/LConn1
  Three-Phase Breaker3/LConn2 -- L824-828a config 301/LConn2
  L824-828a config 301/LConn3 -- Three-Phase Breaker3/LConn3
  824/LConn3 -- Three-Phase Breaker3/RConn1
  824/LConn1 -- Three-Phase Breaker3/RConn3
  Load Flow Bar1/RConn3 -- Three-Phase Breaker1/LConn3
  Load Flow Bar1/RConn2 -- Three-Phase Breaker1/LConn2
  Load Flow Bar1/RConn1 -- Three-Phase Breaker1/LConn1
  Three-Phase Breaker1/RConn1 -- L800-802 config 300/LConn1
  Three-Phase Breaker1/RConn2 -- L800-802 config 300/LConn2
  Three-Phase Breaker1/RConn3 -- L800-802 config 300/LConn3
  Three-Phase Breaker4/LConn2 -- " L808-810a config 303 "/LConn1
